simulink model "V126_L5_UMS"  (R2020b)
settings: Solver=VariableStepAuto  StartTime=0.0  StopTime=200  MaxStep=0.01  RelTol=1e-3
values from neighbouring files (symbols this model uses):
  acs = ap+K*bp    [untitled.m]
  ap = Wp.Denominator{1}    [untitled.m]
  bp = Wp.Numerator{1}    [untitled.m]
  K = 11    [untitled.m]
  K1 = 0.3    [untitled.m]
  K2 = 0.2    [untitled.m]
  mcs = mp+K*np    [untitled.m]
  mp = Wpzoh.Denominator{1}    [untitled.m]
  np = Wpzoh.Numerator{1}    [untitled.m]
  q = 0.3    [untitled.m]
  T1 = 4    [untitled.m]
  T2 = 6    [untitled.m]
  T3 = 0.8    [untitled.m]
  Ts = 0.1* (T1 + T2 + T3)    (= 1.08)    [untitled.m]
  Un = 100    [untitled.m]
settings Model: Creator=td  LastModifiedBy=Maxim
settings DataIOCC: ReturnWorkspaceOutputs=off
settings DebuggingCC: ArithmeticOperatorsInVariantConditions=warning
settings SFSimCC: CustomCodeUndefinedFunction=UseInterfaceOnly

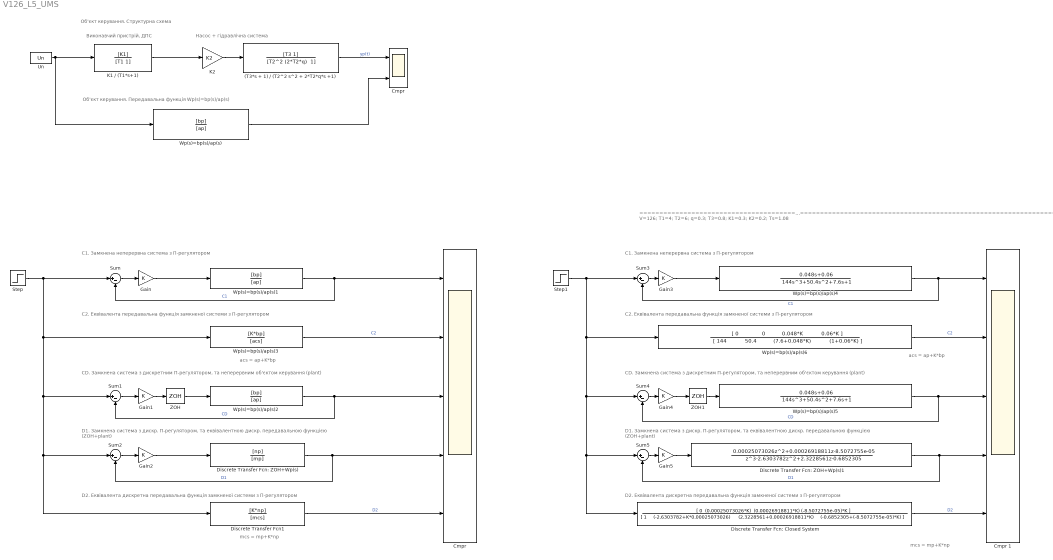
== system V126_L5_UMS ==
  note: =======================================================================================================
      | V=126;  T1=4;  T2=6;  q=0.3;  T3=0.8;  K1=0.3;  K2=0.2;
      | Ts=1.08
  note: acs = ap+K*bp
  note: С1. Замкнена неперервна система з П-регулятором
  note: mcs = mp+K*np
  note: Насос + гідравлічна система
  note: Об'єкт керування. Структурна схема
  note: Виконавчий пристрій, ДПС
  note: Об'єкт керування. Передавальна функція Wp(s)=bp(s)/ap(s)
  note: С2. Еквівалента передавальна функція замкненої системи з П-регулятором
  note: СD. Замкнена система з дискретним П-регулятором, та неперервним об'єктом керування (plant)
  note: D1. Замкнена система з дискр. П-регулятором, та еквівалентною дискр. передавальною функцією (ZOH+plant)
  note: D2. Еквівалента дискретна передавальна функція замкненої системи з П-регулятором
  note: С1. Замкнена неперервна система з П-регулятором
  note: СD. Замкнена система з дискретним П-регулятором, та неперервним об'єктом керування (plant)
  note: С2. Еквівалента передавальна функція замкненої системи з П-регулятором
  note: mcs = mp+K*np
  note: D1. Замкнена система з дискр. П-регулятором, та еквівалентною дискр. передавальною функцією (ZOH+plant)
  note: D2. Еквівалента дискретна передавальна функція замкненої системи з П-регулятором
  note: acs = ap+K*bp
  " Discrete Transfer Fcn: Closed System" : DiscreteTransferFcn  Numerator="[ 0  (0.00025073026*K)  (0.00026918811*K) (-8.5072755e-05)*K ]"  Denominator="[ 1     (-2.6303782+K*0.00025073026)      (2.3228561+0.00026918811*K)     (-0.6852305+(-8.5072755e-05)*K) ]"  SampleTime=Ts
  " Discrete Transfer Fcn: ZOH+Wp(s)" : DiscreteTransferFcn  Numerator=[np]  Denominator=[mp]  SampleTime=Ts
  " Discrete Transfer Fcn: ZOH+Wp(s)1" : DiscreteTransferFcn  Numerator="[ 0  0.00025073026  0.00026918811 -8.5072755e-05 ]"  Denominator="[ 1     -2.6303782      2.3228561     -0.6852305 ]"  SampleTime=Ts
  (T3*s + 1) / (T2^2 s^2 + 2*T2*q*s +1) : TransferFcn  Numerator=[T3 1]  Denominator="[T2^2 (2*T2*q)  1]"
  Cmpr : Scope  NumInputPorts=2
  "Cmpr " : Scope  NumInputPorts=5
  Cmpr 1 : Scope  NumInputPorts=5
  Discrete Transfer Fcn1 : DiscreteTransferFcn  Numerator=[K*np]  Denominator=[mcs]  SampleTime=Ts
  Gain{,1..5} (6 alike) : Gain  Gain=K
  K1 / (T1*s+1) : TransferFcn  Numerator=[K1]  Denominator=[T1 1]
  K2 : Gain  Gain=K2
  Step : Step  SampleTime=0
  Step1 : Step  SampleTime=0
  Sum{,1..5} (6 alike) : Sum  Inputs=|+-
  Un : Constant  Value=Un
  Wp(s)=bp(s)/ap(s) : TransferFcn  Numerator=[bp]  Denominator=[ap]
  Wp(s)=bp(s)/ap(s)1 : TransferFcn  Numerator=[bp]  Denominator=[ap]
  Wp(s)=bp(s)/ap(s)2 : TransferFcn  Numerator=[bp]  Denominator=[ap]
  Wp(s)=bp(s)/ap(s)3 : TransferFcn  Numerator=[K*bp]  Denominator=[acs]
  Wp(s)=bp(s)/ap(s)4 : TransferFcn  Numerator="[ 0              0          0.048           0.06 ]"  Denominator="[ 144           50.4            7.6              1 ]"
  Wp(s)=bp(s)/ap(s)5 : TransferFcn  Numerator="[ 0              0          0.048           0.06 ]"  Denominator="[ 144           50.4            7.6              1 ]"
  Wp(s)=bp(s)/ap(s)6 : TransferFcn  Numerator="[ 0              0          0.048*K           0.06*K ]"  Denominator="[ 144           50.4          (7.6+0.048*K)           (1+0.06*K) ]"
  ZOH : ZeroOrderHold  SampleTime=Ts
  ZOH1 : ZeroOrderHold  SampleTime=Ts
  wires:
  Un/1 -> Wp(s)=bp(s)/ap(s)/1, K1 / (T1*s+1)/1
  K2/1 -> (T3*s + 1) / (T2^2 s^2 + 2*T2*q*s +1)/1
  (T3*s + 1) / (T2^2 s^2 + 2*T2*q*s +1)/1 -> Cmpr/1  "yp(t)"
  K1 / (T1*s+1)/1 -> K2/1
  Wp(s)=bp(s)/ap(s)/1 -> Cmpr/2
  Wp(s)=bp(s)/ap(s)1/1 -> Sum/2, "Cmpr "/1  "C1"
  Wp(s)=bp(s)/ap(s)2/1 -> Sum1/2, "Cmpr "/3  "CD"
  Step/1 -> Sum/1, Sum1/1, Sum2/1, Discrete Transfer Fcn1/1, Wp(s)=bp(s)/ap(s)3/1
  ZOH/1 -> Wp(s)=bp(s)/ap(s)2/1
  Sum/1 -> Gain/1
  Gain/1 -> Wp(s)=bp(s)/ap(s)1/1
  Sum1/1 -> Gain1/1
  Gain1/1 -> ZOH/1
  Gain2/1 -> " Discrete Transfer Fcn: ZOH+Wp(s)"/1
  Sum2/1 -> Gain2/1
  " Discrete Transfer Fcn: ZOH+Wp(s)"/1 -> Sum2/2, "Cmpr "/4  "D1"
  Wp(s)=bp(s)/ap(s)3/1 -> "Cmpr "/2  "C2"
  Discrete Transfer Fcn1/1 -> "Cmpr "/5  "D2"
  Wp(s)=bp(s)/ap(s)5/1 -> Cmpr 1/3, Sum4/2  "CD"
  " Discrete Transfer Fcn: ZOH+Wp(s)1"/1 -> Sum5/2, Cmpr 1/4  "D1"
  Gain4/1 -> ZOH1/1
  Sum3/1 -> Gain3/1
  Gain3/1 -> Wp(s)=bp(s)/ap(s)4/1
  Wp(s)=bp(s)/ap(s)6/1 -> Cmpr 1/2  "C2"
  Sum4/1 -> Gain4/1
  Gain5/1 -> " Discrete Transfer Fcn: ZOH+Wp(s)1"/1
  Wp(s)=bp(s)/ap(s)4/1 -> Sum3/2, Cmpr 1/1  "C1"
  Step1/1 -> " Discrete Transfer Fcn: Closed System"/1, Sum5/1, Sum4/1, Wp(s)=bp(s)/ap(s)6/1, Sum3/1
  Sum5/1 -> Gain5/1
  ZOH1/1 -> Wp(s)=bp(s)/ap(s)5/1
  " Discrete Transfer Fcn: Closed System"/1 -> Cmpr 1/5  "D2"
